simulink model "MG2Controller_TestHarness"  (R2021a)
settings: Solver=VariableStepAuto  StartTime=0.0  StopTime=10.0  RelTol=1e-3
PreLoadFcn:
  | MG2Controller_Setup
settings Model: Creator=isaacito  LastModifiedBy=isaacito

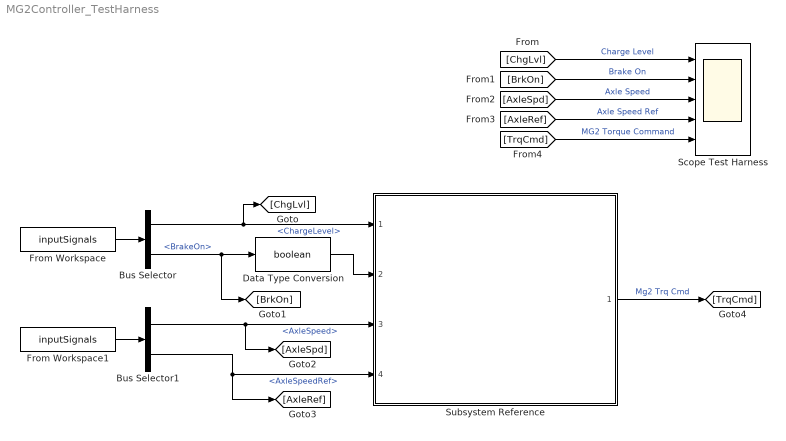
== system MG2Controller_TestHarness ==
  Bus Selector : BusSelector  OutputSignals=ChargeLevel,BrakeOn
  Bus Selector1 : BusSelector  OutputSignals=AxleSpeed,AxleSpeedRef
  Data Type Conversion : DataTypeConversion  OutDataTypeStr=boolean
  From Workspace : FromWorkspace  VariableName=inputSignals  OutDataTypeStr=Bus: inputBus  Interpolate=off  OutputAfterFinalValue=Holding final value
      settings: AttributesFormatString=|
      | %<OutDataTypeStr>
      | Interpolate: %<Interpolate>
  From Workspace1 : FromWorkspace  VariableName=inputSignals  OutDataTypeStr=Bus: inputBus  OutputAfterFinalValue=Holding final value
      settings: AttributesFormatString=|
      | %<OutDataTypeStr>
      | Interpolate: %<Interpolate>
  Scope Test Harness : Scope  NumInputPorts=5
  Subsystem Reference : Subsystem  ReferencedSubsystem=MG2Controller_HEVPowerSplit_refsub
  wires:
  From Workspace/1 -> Bus Selector/1
  Bus Selector/1 -> [ChgLvl], Subsystem Reference/1  "<ChargeLevel>"
  Bus Selector/2 -> [BrkOn], Data Type Conversion/1  "<BrakeOn>"
  From Workspace1/1 -> Bus Selector1/1
  Bus Selector1/1 -> [AxleSpd], Subsystem Reference/3  "<AxleSpeed>"
  Bus Selector1/2 -> [AxleRef], Subsystem Reference/4  "<AxleSpeedRef>"
  Subsystem Reference/1 -> [TrqCmd]  "Mg2 Trq Cmd"
  Data Type Conversion/1 -> Subsystem Reference/2
  [ChgLvl] -> Scope Test Harness/1  "Charge Level"
  [BrkOn] -> Scope Test Harness/2  "Brake On"
  [AxleSpd] -> Scope Test Harness/3  "Axle Speed"
  [AxleRef] -> Scope Test Harness/4  "Axle Speed Ref"
  [TrqCmd] -> Scope Test Harness/5  "MG2 Torque Command"
